simulink model "exampl_smlk"  (R2021b)
settings: Solver=VariableStepAuto  StartTime=0.0  StopTime=10.0  RelTol=1e-3
values from neighbouring files (symbols this model uses):
  C0 = 1/(C*Ce*(tauC+L/2))    (= 4.44444444444)    [Paramaeters.m]
  C1 = max(T,L/2)*C0    [Paramaeters.m]
  Cd = min(T,L/2)*Ce    [Paramaeters.m]
  Ce = 1    [Paramaeters.m]
libraries: fuzblock x1
settings Model: Creator=Mazou  LastModifiedBy=Mazou

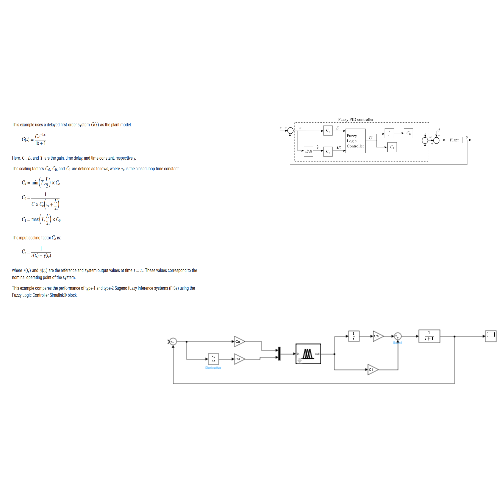
[thumbnail: Simulink's stored preview of the top-level diagram]
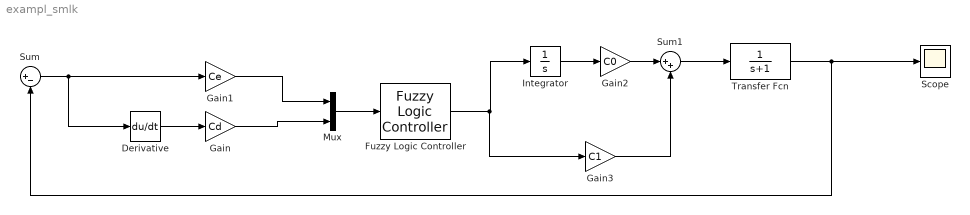
== system exampl_smlk ==
  Derivative : Derivative
  Fuzzy Logic Controller : fuzblock/Fuzzy Logic  Controller  FIS='tipper.fis'  OutputSampleNumber=101  DataType=double  FuzzifiedInputs=off  RuleFiringStrengths=off  RuleOutputs=off  AggregatedOutputs=off  SimulateUsing=Interpreted execution  OutOfRangeInputValueMessage=warning  NoRuleFiredMessage=warning  EmptyOutputFuzzySetMessage=warning
  Gain : Gain  Gain=Cd
  Gain1 : Gain  Gain=Ce
  Gain2 : Gain  Gain=C0
  Gain3 : Gain  Gain=C1
  Integrator : Integrator
  Mux : Mux  Inputs=2
  Scope : Scope
  Sum : Sum  Inputs=|+-
  Sum1 : Sum  Inputs=|++
  Transfer Fcn : TransferFcn  Denominator=[1 1]
  wires:
  Mux/1 -> Fuzzy Logic Controller/1
  Gain/1 -> Mux/2
  Gain1/1 -> Mux/1
  Integrator/1 -> Gain2/1
  Fuzzy Logic Controller/1 -> Gain3/1, Integrator/1
  Derivative/1 -> Gain/1
  Sum/1 -> Derivative/1, Gain1/1
  Transfer Fcn/1 -> Sum/2, Scope/1
  Gain3/1 -> Sum1/2
  Gain2/1 -> Sum1/1
  Sum1/1 -> Transfer Fcn/1
